simulink model "vdp_100"  (R2023b)
settings: Solver=VariableStepAuto  StartTime=0.0  StopTime=20  RelTol=1e-3  AbsTol=1e-6
libraries: simulink x100
(part 1 of 2)
Description:
  | The van der Pol Equation
  | 
  | This is a simulation of a nonlinear second order system.
settings Model: Creator=The MathWorks, Inc.  LastModifiedBy=dganesan
settings SolverCC: AutoScaleAbsTol=off  AlgebraicLoopSolver=TrustRegion
settings DataIOCC: ExternalInput=[]  InitialState=[]  SaveFormat=Array  SaveOutput=off  SaveTime=off
settings OptimizationCC: BlockReduction=off  BooleanDataType=off  ReuseModelBlockBuffer=off  InitFltsAndDblsToZero=on  LifeSpan=inf  BufferReusableBoundary=off
settings DebuggingCC: SaveWithParameterizedLinksMsg=none  SignalResolutionControl=TryResolveAllWithWarning  MultiTaskDSMMsg=warning  MultiTaskCondExecSysMsg=none  FcnCallInpInsideContextMsg=warning  UnconnectedInputMsg=warning  UnconnectedOutputMsg=warning  UnconnectedLineMsg=warning  BusObjectLabelMismatch=none  PregeneratedLibrarySubsystemCodeDiagnostic=none  SFUnexpectedBacktrackingDiag=warning  SFNoUnconditionalDefaultTransitionDiag=warning  SFExecutionAtInitializationDiag=none  ArithmeticOperatorsInVariantConditions=warning
settings HardwareCC: ProdBitPerPointer=32  ProdBitPerSizeT=32  ProdBitPerPtrDiffT=32  ProdLargestAtomicFloat=None  ProdIntDivRoundTo=Undefined  ProdEndianess=Unspecified  ProdWordSize=32  ProdHWDeviceType=32-bit Generic  TargetUnknown=on
settings ModelReferenceCC: EnableRefExpFcnMdlSchedulingChecks=on  PropagateSignalLabelsOutOfModel=off
settings SFSimCC: SimUseLocalCustomCode=off  CustomCodeUndefinedFunction=UseInterfaceOnly
settings RTWCC: RTWUseLocalCustomCode=off
settings CodeAppCC: StateflowObjectComments=on
settings GRTTargetCC: TargetFcnLib=ansi_tfl_tmw.mat  TargetLangStandard=C89/C90 (ANSI)  CombineOutputUpdateFcns=off  GRTInterface=on
settings ConfigComp: CovMetricSettings=dw  CovSaveCumulativeToWorkspaceVar=on  CovSaveSingleToWorkspaceVar=on  CovExternalEMLEnable=off

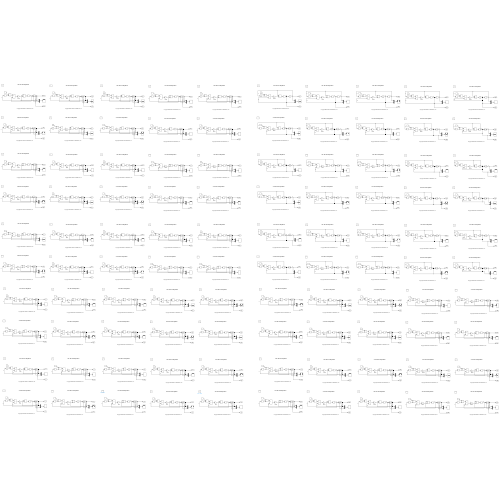
[thumbnail: Simulink's stored preview of the top-level diagram]
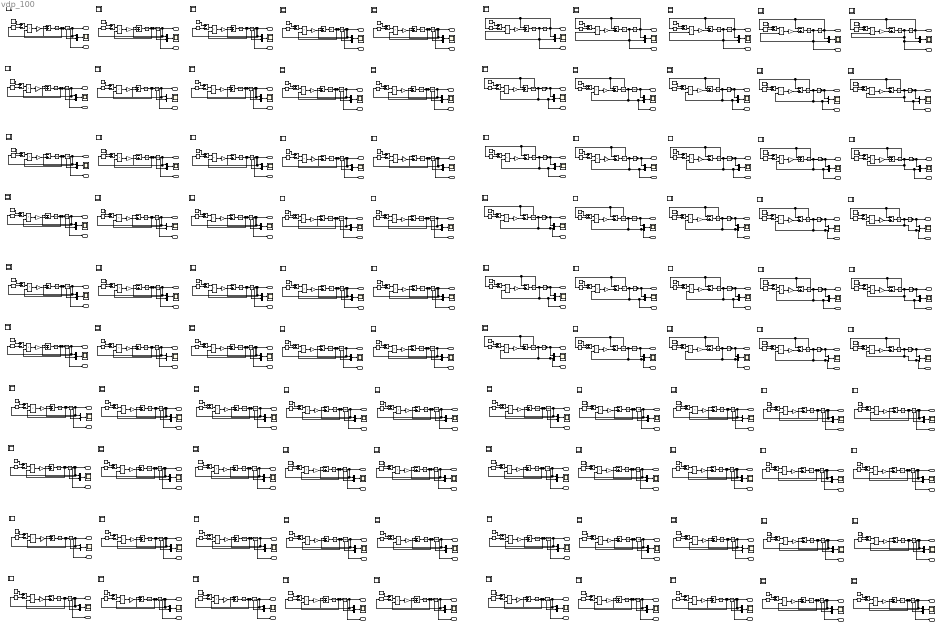
== system vdp_100 ==
  note: van der Pol Equation
  note: Copyright 2004-2020 The MathWorks, Inc.
  note: van der Pol Equation
  note: Copyright 2004-2020 The MathWorks, Inc.
  note: van der Pol Equation
  note: Copyright 2004-2020 The MathWorks, Inc.
  note: Copyright 2004-2020 The MathWorks, Inc.
  note: van der Pol Equation
  note: Copyright 2004-2020 The MathWorks, Inc.
  note: van der Pol Equation
  note: van der Pol Equation
  note: Copyright 2004-2020 The MathWorks, Inc.
  note: van der Pol Equation
  note: van der Pol Equation
  note: Copyright 2004-2020 The MathWorks, Inc.
  note: Copyright 2004-2020 The MathWorks, Inc.
  note: Copyright 2004-2020 The MathWorks, Inc.
  note: Copyright 2004-2020 The MathWorks, Inc.
  note: van der Pol Equation
  note: van der Pol Equation
  note: van der Pol Equation
  note: Copyright 2004-2020 The MathWorks, Inc.
  note: van der Pol Equation
  note: Copyright 2004-2020 The MathWorks, Inc.
  note: Copyright 2004-2020 The MathWorks, Inc.
  note: van der Pol Equation
  note: Copyright 2004-2020 The MathWorks, Inc.
  note: van der Pol Equation
  note: Copyright 2004-2020 The MathWorks, Inc.
  note: Copyright 2004-2020 The MathWorks, Inc.
  note: van der Pol Equation
  note: van der Pol Equation
  note: van der Pol Equation
  note: van der Pol Equation
  note: Copyright 2004-2020 The MathWorks, Inc.
  note: Copyright 2004-2020 The MathWorks, Inc.
  note: Copyright 2004-2020 The MathWorks, Inc.
  note: Copyright 2004-2020 The MathWorks, Inc.
  note: van der Pol Equation
  note: van der Pol Equation
  note: van der Pol Equation
  note: Copyright 2004-2020 The MathWorks, Inc.
  note: van der Pol Equation
  note: Copyright 2004-2020 The MathWorks, Inc.
  note: van der Pol Equation
  note: Copyright 2004-2020 The MathWorks, Inc.
  note: van der Pol Equation
  note: van der Pol Equation
  note: van der Pol Equation
  note: van der Pol Equation
  note: Copyright 2004-2020 The MathWorks, Inc.
  note: van der Pol Equation
  note: Copyright 2004-2020 The MathWorks, Inc.
  note: van der Pol Equation
  note: Copyright 2004-2020 The MathWorks, Inc.
  note: Copyright 2004-2020 The MathWorks, Inc.
  note: Copyright 2004-2020 The MathWorks, Inc.
  note: Copyright 2004-2020 The MathWorks, Inc.
  note: Copyright 2004-2020 The MathWorks, Inc.
  note: van der Pol Equation
  note: van der Pol Equation
  note: Copyright 2004-2020 The MathWorks, Inc.
  note: Copyright 2004-2020 The MathWorks, Inc.
  note: van der Pol Equation
  note: Copyright 2004-2020 The MathWorks, Inc.
  note: van der Pol Equation
  note: Copyright 2004-2020 The MathWorks, Inc.
  note: van der Pol Equation
  note: Copyright 2004-2020 The MathWorks, Inc.
  note: Copyright 2004-2020 The MathWorks, Inc.
  note: van der Pol Equation
  note: van der Pol Equation
  note: van der Pol Equation
  note: van der Pol Equation
  note: Copyright 2004-2020 The MathWorks, Inc.
  note: Copyright 2004-2020 The MathWorks, Inc.
  note: Copyright 2004-2020 The MathWorks, Inc.
  note: Copyright 2004-2020 The MathWorks, Inc.
  note: van der Pol Equation
  note: van der Pol Equation
  note: van der Pol Equation
  note: Copyright 2004-2020 The MathWorks, Inc.
  note: Copyright 2004-2020 The MathWorks, Inc.
  note: Copyright 2004-2020 The MathWorks, Inc.
  note: van der Pol Equation
  note: Copyright 2004-2020 The MathWorks, Inc.
  note: van der Pol Equation
  note: Copyright 2004-2020 The MathWorks, Inc.
  note: van der Pol Equation
  note: Copyright 2004-2020 The MathWorks, Inc.
  note: Copyright 2004-2020 The MathWorks, Inc.
  note: van der Pol Equation
  note: van der Pol Equation
  note: Copyright 2004-2020 The MathWorks, Inc.
  note: Copyright 2004-2020 The MathWorks, Inc.
  note: Copyright 2004-2020 The MathWorks, Inc.
  note: van der Pol Equation
  note: van der Pol Equation
  note: van der Pol Equation
  note: van der Pol Equation
  note: Copyright 2004-2020 The MathWorks, Inc.
  note: van der Pol Equation
  note: van der Pol Equation
  note: Copyright 2004-2020 The MathWorks, Inc.
  note: van der Pol Equation
  note: Copyright 2004-2020 The MathWorks, Inc.
  note: Copyright 2004-2020 The MathWorks, Inc.
  note: Copyright 2004-2020 The MathWorks, Inc.
  note: Copyright 2004-2020 The MathWorks, Inc.
  note: van der Pol Equation
  note: van der Pol Equation
  note: Copyright 2004-2020 The MathWorks, Inc.
  note: van der Pol Equation
  note: van der Pol Equation
  note: Copyright 2004-2020 The MathWorks, Inc.
  note: van der Pol Equation
  note: Copyright 2004-2020 The MathWorks, Inc.
  note: van der Pol Equation
  note: Copyright 2004-2020 The MathWorks, Inc.
  note: van der Pol Equation
  note: van der Pol Equation
  note: van der Pol Equation
  note: Copyright 2004-2020 The MathWorks, Inc.
  note: van der Pol Equation
  note: van der Pol Equation
  note: Copyright 2004-2020 The MathWorks, Inc.
  note: Copyright 2004-2020 The MathWorks, Inc.
  note: Copyright 2004-2020 The MathWorks, Inc.
  note: van der Pol Equation
  note: van der Pol Equation
  note: van der Pol Equation
  note: Copyright 2004-2020 The MathWorks, Inc.
  note: Copyright 2004-2020 The MathWorks, Inc.
  note: Copyright 2004-2020 The MathWorks, Inc.
  note: Copyright 2004-2020 The MathWorks, Inc.
  note: van der Pol Equation
  note: Copyright 2004-2020 The MathWorks, Inc.
  note: Copyright 2004-2020 The MathWorks, Inc.
  note: Copyright 2004-2020 The MathWorks, Inc.
  note: van der Pol Equation
  note: van der Pol Equation
  note: van der Pol Equation
  note: Copyright 2004-2020 The MathWorks, Inc.
  note: van der Pol Equation
  note: van der Pol Equation
  note: van der Pol Equation
  note: van der Pol Equation
  note: Copyright 2004-2020 The MathWorks, Inc.
  note: Copyright 2004-2020 The MathWorks, Inc.
  note: van der Pol Equation
  note: van der Pol Equation
  note: Copyright 2004-2020 The MathWorks, Inc.
  note: van der Pol Equation
  note: Copyright 2004-2020 The MathWorks, Inc.
  note: van der Pol Equation
  note: van der Pol Equation
  note: van der Pol Equation
  note: van der Pol Equation
  note: van der Pol Equation
  note: Copyright 2004-2020 The MathWorks, Inc.
  note: Copyright 2004-2020 The MathWorks, Inc.
  note: van der Pol Equation
  note: Copyright 2004-2020 The MathWorks, Inc.
  note: van der Pol Equation
  note: Copyright 2004-2020 The MathWorks, Inc.
  note: Copyright 2004-2020 The MathWorks, Inc.
  note: Copyright 2004-2020 The MathWorks, Inc.
  note: Copyright 2004-2020 The MathWorks, Inc.
  note: Copyright 2004-2020 The MathWorks, Inc.
  note: van der Pol Equation
  note: Copyright 2004-2020 The MathWorks, Inc.
  note: Copyright 2004-2020 The MathWorks, Inc.
  note: van der Pol Equation
  note: Copyright 2004-2020 The MathWorks, Inc.
  note: van der Pol Equation
  note: Copyright 2004-2020 The MathWorks, Inc.
  note: van der Pol Equation
  note: van der Pol Equation
  note: van der Pol Equation
  note: Copyright 2004-2020 The MathWorks, Inc.
  note: van der Pol Equation
  note: Copyright 2004-2020 The MathWorks, Inc.
  note: Copyright 2004-2020 The MathWorks, Inc.
  note: van der Pol Equation
  note: Copyright 2004-2020 The MathWorks, Inc.
  note: Copyright 2004-2020 The MathWorks, Inc.
  note: van der Pol Equation
  note: Copyright 2004-2020 The MathWorks, Inc.
  note: van der Pol Equation
  note: van der Pol Equation
  note: van der Pol Equation
  note: Copyright 2004-2020 The MathWorks, Inc.
  note: Copyright 2004-2020 The MathWorks, Inc.
  note: Copyright 2004-2020 The MathWorks, Inc.
  note: van der Pol Equation
  note: Copyright 2004-2020 The MathWorks, Inc.
  note: Copyright 2004-2020 The MathWorks, Inc.
  note: Copyright 2004-2020 The MathWorks, Inc.
  note: van der Pol Equation
  note: van der Pol Equation
  Constant{,1..99} (100 alike) : Constant
  More Info : Subsystem
      mask Display: disp('?')
  More Info1 : Subsystem
      mask Display: disp('?')
  More Info10 : Subsystem
      mask Display: disp('?')
  More Info11 : Subsystem
      mask Display: disp('?')
  More Info12 : Subsystem
      mask Display: disp('?')
  More Info13 : Subsystem
      mask Display: disp('?')
  More Info14 : Subsystem
      mask Display: disp('?')
  More Info15 : Subsystem
      mask Display: disp('?')
  More Info16 : Subsystem
      mask Display: disp('?')
  More Info17 : Subsystem
      mask Display: disp('?')
  More Info18 : Subsystem
      mask Display: disp('?')
  More Info19 : Subsystem
      mask Display: disp('?')
  More Info2 : Subsystem
      mask Display: disp('?')
  More Info20 : Subsystem
      mask Display: disp('?')
  More Info21 : Subsystem
      mask Display: disp('?')
  More Info22 : Subsystem
      mask Display: disp('?')
  More Info23 : Subsystem
      mask Display: disp('?')
  More Info24 : Subsystem
      mask Display: disp('?')
  More Info25 : Subsystem
      mask Display: disp('?')
  More Info26 : Subsystem
      mask Display: disp('?')
  More Info27 : Subsystem
      mask Display: disp('?')
  More Info28 : Subsystem
      mask Display: disp('?')
  More Info29 : Subsystem
      mask Display: disp('?')
  More Info3 : Subsystem
      mask Display: disp('?')
  More Info30 : Subsystem
      mask Display: disp('?')
  More Info31 : Subsystem
      mask Display: disp('?')
  More Info32 : Subsystem
      mask Display: disp('?')
  More Info33 : Subsystem
      mask Display: disp('?')
  More Info34 : Subsystem
      mask Display: disp('?')
  More Info35 : Subsystem
      mask Display: disp('?')
  More Info36 : Subsystem
      mask Display: disp('?')
  More Info37 : Subsystem
      mask Display: disp('?')
  More Info38 : Subsystem
      mask Display: disp('?')
  More Info39 : Subsystem
      mask Display: disp('?')
  More Info4 : Subsystem
      mask Display: disp('?')
  More Info40 : Subsystem
      mask Display: disp('?')
  More Info41 : Subsystem
      mask Display: disp('?')
  More Info42 : Subsystem
      mask Display: disp('?')
  More Info43 : Subsystem
      mask Display: disp('?')
  More Info44 : Subsystem
      mask Display: disp('?')
  More Info45 : Subsystem
      mask Display: disp('?')
  More Info46 : Subsystem
      mask Display: disp('?')
  More Info47 : Subsystem
      mask Display: disp('?')
  More Info48 : Subsystem
      mask Display: disp('?')
  More Info49 : Subsystem
      mask Display: disp('?')
  More Info5 : Subsystem
      mask Display: disp('?')
  More Info50 : Subsystem
      mask Display: disp('?')
  More Info51 : Subsystem
      mask Display: disp('?')
  More Info52 : Subsystem
      mask Display: disp('?')
  More Info53 : Subsystem
      mask Display: disp('?')
  More Info54 : Subsystem
      mask Display: disp('?')
  More Info55 : Subsystem
      mask Display: disp('?')
  More Info56 : Subsystem
      mask Display: disp('?')
  More Info57 : Subsystem
      mask Display: disp('?')
  More Info58 : Subsystem
      mask Display: disp('?')
  More Info59 : Subsystem
      mask Display: disp('?')
  More Info6 : Subsystem
      mask Display: disp('?')
  More Info60 : Subsystem
      mask Display: disp('?')
  More Info61 : Subsystem
      mask Display: disp('?')
  More Info62 : Subsystem
      mask Display: disp('?')
  More Info63 : Subsystem
      mask Display: disp('?')
  More Info64 : Subsystem
      mask Display: disp('?')
  More Info65 : Subsystem
      mask Display: disp('?')
  More Info66 : Subsystem
      mask Display: disp('?')
  More Info67 : Subsystem
      mask Display: disp('?')
  More Info68 : Subsystem
      mask Display: disp('?')
  More Info69 : Subsystem
      mask Display: disp('?')
  More Info7 : Subsystem
      mask Display: disp('?')
  More Info70 : Subsystem
      mask Display: disp('?')
  More Info71 : Subsystem
      mask Display: disp('?')
  More Info72 : Subsystem
      mask Display: disp('?')
  More Info73 : Subsystem
      mask Display: disp('?')
  More Info74 : Subsystem
      mask Display: disp('?')
  More Info75 : Subsystem
      mask Display: disp('?')
  More Info76 : Subsystem
      mask Display: disp('?')
  More Info77 : Subsystem
      mask Display: disp('?')
  More Info78 : Subsystem
      mask Display: disp('?')
  More Info79 : Subsystem
      mask Display: disp('?')
  More Info8 : Subsystem
      mask Display: disp('?')
  More Info80 : Subsystem
      mask Display: disp('?')
  More Info81 : Subsystem
      mask Display: disp('?')
  More Info82 : Subsystem
      mask Display: disp('?')
  More Info83 : Subsystem
      mask Display: disp('?')
  More Info84 : Subsystem
      mask Display: disp('?')
  More Info85 : Subsystem
      mask Display: disp('?')
  More Info86 : Subsystem
      mask Display: disp('?')
  More Info87 : Subsystem
      mask Display: disp('?')
  More Info88 : Subsystem
      mask Display: disp('?')
  More Info89 : Subsystem
      mask Display: disp('?')
  More Info9 : Subsystem
      mask Display: disp('?')
  More Info90 : Subsystem
      mask Display: disp('?')
  More Info91 : Subsystem
      mask Display: disp('?')
  More Info92 : Subsystem
      mask Display: disp('?')
  More Info93 : Subsystem
      mask Display: disp('?')
  More Info94 : Subsystem
      mask Display: disp('?')
  More Info95 : Subsystem
      mask Display: disp('?')
  More Info96 : Subsystem
      mask Display: disp('?')
  More Info97 : Subsystem
      mask Display: disp('?')
  More Info98 : Subsystem
      mask Display: disp('?')
  More Info99 : Subsystem
      mask Display: disp('?')
  Mu{,1..99} (100 alike) : Gain  SaturateOnIntegerOverflow=on  OutDataTypeStr=Inherit: Same as input  ParamDataTypeStr=Inherit: Same as input
  Mux{,1..99} (100 alike) : Mux  Inputs=2
  Product{,1..99} (100 alike) : Product  InputSameDT=on  RndMeth=Zero  SaturateOnIntegerOverflow=on  OutDataTypeStr=Inherit: Same as first input
  Scope{,1..99} (100 alike) : Scope
  Square{,1..99} (100 alike) : Math  Operator=square
  Sum{,2,4,6,8,10,12,14,16,18,20,22,24,26,28,30,32,34,36,38,40,42,44,46,48,50,52..53,55,57,59,61,64,66,68,70,72,74,76,78,80,82,84,86,88,90,92,94,96,98,100,102,104,106,108,110,112..113,115,117,119,121,124,126,128,130,132,134..135,137,139,141,143,146,148..149,151,153,155..156,158,161,163,165,168,170,172,174,176,178..179,181,183,185,187,190,192,194,196,198} (100 alike) : Sum  Inputs=-+  InputSameDT=on  SaturateOnIntegerOverflow=on  OutDataTypeStr=Inherit: Same as first input
  Sum{1,3,5,7,9,11,13,15,17,19,21,23,25,27,29,31,33,35,37,39,41,43,45,47,49,51,54,56,58,60,62..63,65,67,69,71,73,75,77,79,81,83,85,87,89,91,93,95,97,99,101,103,105,107,109,111,114,116,118,120,122..123,125,127,129,131,133,136,138,140,142,144..145,147,150,152,154,157,159..160,162,164,166..167,169,171,173,175,177,180,182,184,186,188..189,191,193,195,197,199} (100 alike) : Sum  Inputs=+-  InputSameDT=on  SaturateOnIntegerOverflow=on  OutDataTypeStr=Inherit: Same as first input
  x{1,3,5,7,9,11,14,16,18,20..21,23,26,28,30,33..34,36,38,40..41,43,46,48,50,53..54,56,59,61,63..64,67..68,70,72,75..76,78,80..81,83,86,88,90,93..94,96,98,100..101,103..104,107,109,111,114..115,117,120,122,124..125,128..129,131,133,136..137,139,142,144,146..147,150..151,153,156,159,161..162,165..166,168..169,171,174..175,177,180..181,183,186,188,190..191,194..195,197,199} (100 alike) : Integrator  InitialCondition=2
  x{2,4,6,8,10,12..13,15,17,19,22,24..25,27,29,31..32,35,37,39,42,44..45,47,49,51..52,55,57..58,60,62,65..66,69,71,73..74,77,79,82,84..85,87,89,91..92,95,97,99,102,105..106,108,110,112..113,116,118..119,121,123,126..127,130,132,134..135,138,140..141,143,145,148..149,152,154..155,157..158,160,163..164,167,170,172..173,176,178..179,182,184..185,187,189,192..193,196,198,200} (100 alike) : Integrator
  Out1 : Outport  InitialOutput=0  VectorParamsAs1DForOutWhenUnconnected=off
  Out2 : Outport  Port=2  InitialOutput=0  VectorParamsAs1DForOutWhenUnconnected=off
  Out3 : Outport  Port=3  InitialOutput=0  VectorParamsAs1DForOutWhenUnconnected=off
  Out4 : Outport  Port=4  InitialOutput=0  VectorParamsAs1DForOutWhenUnconnected=off
  Out5 : Outport  Port=5  InitialOutput=0  VectorParamsAs1DForOutWhenUnconnected=off
  Out6 : Outport  Port=6  InitialOutput=0  VectorParamsAs1DForOutWhenUnconnected=off
  Out7 : Outport  Port=7  InitialOutput=0  VectorParamsAs1DForOutWhenUnconnected=off
  Out8 : Outport  Port=8  InitialOutput=0  VectorParamsAs1DForOutWhenUnconnected=off
  Out9 : Outport  Port=9  InitialOutput=0  VectorParamsAs1DForOutWhenUnconnected=off
  Out10 : Outport  Port=10  InitialOutput=0  VectorParamsAs1DForOutWhenUnconnected=off
  Out11 : Outport  Port=11  InitialOutput=0  VectorParamsAs1DForOutWhenUnconnected=off
  Out12 : Outport  Port=12  InitialOutput=0  VectorParamsAs1DForOutWhenUnconnected=off
  Out13 : Outport  Port=13  InitialOutput=0  VectorParamsAs1DForOutWhenUnconnected=off
  Out14 : Outport  Port=14  InitialOutput=0  VectorParamsAs1DForOutWhenUnconnected=off
  Out15 : Outport  Port=15  InitialOutput=0  VectorParamsAs1DForOutWhenUnconnected=off
  Out16 : Outport  Port=16  InitialOutput=0  VectorParamsAs1DForOutWhenUnconnected=off
  Out17 : Outport  Port=17  InitialOutput=0  VectorParamsAs1DForOutWhenUnconnected=off
  Out18 : Outport  Port=18  InitialOutput=0  VectorParamsAs1DForOutWhenUnconnected=off
  Out19 : Outport  Port=19  InitialOutput=0  VectorParamsAs1DForOutWhenUnconnected=off
  Out20 : Outport  Port=20  InitialOutput=0  VectorParamsAs1DForOutWhenUnconnected=off
  Out21 : Outport  Port=21  InitialOutput=0  VectorParamsAs1DForOutWhenUnconnected=off
  Out22 : Outport  Port=22  InitialOutput=0  VectorParamsAs1DForOutWhenUnconnected=off
  Out23 : Outport  Port=23  InitialOutput=0  VectorParamsAs1DForOutWhenUnconnected=off
  Out24 : Outport  Port=24  InitialOutput=0  VectorParamsAs1DForOutWhenUnconnected=off
  Out25 : Outport  Port=25  InitialOutput=0  VectorParamsAs1DForOutWhenUnconnected=off
  Out26 : Outport  Port=26  InitialOutput=0  VectorParamsAs1DForOutWhenUnconnected=off
  Out27 : Outport  Port=27  InitialOutput=0  VectorParamsAs1DForOutWhenUnconnected=off
  Out28 : Outport  Port=28  InitialOutput=0  VectorParamsAs1DForOutWhenUnconnected=off
  Out29 : Outport  Port=29  InitialOutput=0  VectorParamsAs1DForOutWhenUnconnected=off
  Out30 : Outport  Port=30  InitialOutput=0  VectorParamsAs1DForOutWhenUnconnected=off
  Out31 : Outport  Port=31  InitialOutput=0  VectorParamsAs1DForOutWhenUnconnected=off
  Out32 : Outport  Port=32  InitialOutput=0  VectorParamsAs1DForOutWhenUnconnected=off
  Out33 : Outport  Port=33  InitialOutput=0  VectorParamsAs1DForOutWhenUnconnected=off
  Out34 : Outport  Port=34  InitialOutput=0  VectorParamsAs1DForOutWhenUnconnected=off
  Out35 : Outport  Port=35  InitialOutput=0  VectorParamsAs1DForOutWhenUnconnected=off
  Out36 : Outport  Port=36  InitialOutput=0  VectorParamsAs1DForOutWhenUnconnected=off
  Out37 : Outport  Port=37  InitialOutput=0  VectorParamsAs1DForOutWhenUnconnected=off
  Out38 : Outport  Port=38  InitialOutput=0  VectorParamsAs1DForOutWhenUnconnected=off
  Out39 : Outport  Port=39  InitialOutput=0  VectorParamsAs1DForOutWhenUnconnected=off
  Out40 : Outport  Port=40  InitialOutput=0  VectorParamsAs1DForOutWhenUnconnected=off
  Out41 : Outport  Port=41  InitialOutput=0  VectorParamsAs1DForOutWhenUnconnected=off
  Out42 : Outport  Port=42  InitialOutput=0  VectorParamsAs1DForOutWhenUnconnected=off
  Out43 : Outport  Port=43  InitialOutput=0  VectorParamsAs1DForOutWhenUnconnected=off
  Out44 : Outport  Port=44  InitialOutput=0  VectorParamsAs1DForOutWhenUnconnected=off
  Out45 : Outport  Port=45  InitialOutput=0  VectorParamsAs1DForOutWhenUnconnected=off
  Out46 : Outport  Port=46  InitialOutput=0  VectorParamsAs1DForOutWhenUnconnected=off
  Out47 : Outport  Port=47  InitialOutput=0  VectorParamsAs1DForOutWhenUnconnected=off
  Out48 : Outport  Port=48  InitialOutput=0  VectorParamsAs1DForOutWhenUnconnected=off
  Out49 : Outport  Port=49  InitialOutput=0  VectorParamsAs1DForOutWhenUnconnected=off
  Out50 : Outport  Port=50  InitialOutput=0  VectorParamsAs1DForOutWhenUnconnected=off
  Out51 : Outport  Port=51  InitialOutput=0  VectorParamsAs1DForOutWhenUnconnected=off
  Out52 : Outport  Port=52  InitialOutput=0  VectorParamsAs1DForOutWhenUnconnected=off
  Out53 : Outport  Port=53  InitialOutput=0  VectorParamsAs1DForOutWhenUnconnected=off
  Out54 : Outport  Port=54  InitialOutput=0  VectorParamsAs1DForOutWhenUnconnected=off
  Out55 : Outport  Port=55  InitialOutput=0  VectorParamsAs1DForOutWhenUnconnected=off
  Out56 : Outport  Port=56  InitialOutput=0  VectorParamsAs1DForOutWhenUnconnected=off
  Out57 : Outport  Port=57  InitialOutput=0  VectorParamsAs1DForOutWhenUnconnected=off
  Out58 : Outport  Port=58  InitialOutput=0  VectorParamsAs1DForOutWhenUnconnected=off
  Out59 : Outport  Port=59  InitialOutput=0  VectorParamsAs1DForOutWhenUnconnected=off
  Out60 : Outport  Port=60  InitialOutput=0  VectorParamsAs1DForOutWhenUnconnected=off
  Out61 : Outport  Port=61  InitialOutput=0  VectorParamsAs1DForOutWhenUnconnected=off
  Out62 : Outport  Port=62  InitialOutput=0  VectorParamsAs1DForOutWhenUnconnected=off
  Out63 : Outport  Port=63  InitialOutput=0  VectorParamsAs1DForOutWhenUnconnected=off
  Out64 : Outport  Port=64  InitialOutput=0  VectorParamsAs1DForOutWhenUnconnected=off
  Out65 : Outport  Port=65  InitialOutput=0  VectorParamsAs1DForOutWhenUnconnected=off
  Out66 : Outport  Port=66  InitialOutput=0  VectorParamsAs1DForOutWhenUnconnected=off
  Out67 : Outport  Port=67  InitialOutput=0  VectorParamsAs1DForOutWhenUnconnected=off
  Out68 : Outport  Port=68  InitialOutput=0  VectorParamsAs1DForOutWhenUnconnected=off
  Out69 : Outport  Port=69  InitialOutput=0  VectorParamsAs1DForOutWhenUnconnected=off
  Out70 : Outport  Port=70  InitialOutput=0  VectorParamsAs1DForOutWhenUnconnected=off
  Out71 : Outport  Port=71  InitialOutput=0  VectorParamsAs1DForOutWhenUnconnected=off
  Out72 : Outport  Port=72  InitialOutput=0  VectorParamsAs1DForOutWhenUnconnected=off
  Out73 : Outport  Port=73  InitialOutput=0  VectorParamsAs1DForOutWhenUnconnected=off
  Out74 : Outport  Port=74  InitialOutput=0  VectorParamsAs1DForOutWhenUnconnected=off
  Out75 : Outport  Port=75  InitialOutput=0  VectorParamsAs1DForOutWhenUnconnected=off
  Out76 : Outport  Port=76  InitialOutput=0  VectorParamsAs1DForOutWhenUnconnected=off
  Out77 : Outport  Port=77  InitialOutput=0  VectorParamsAs1DForOutWhenUnconnected=off
  Out78 : Outport  Port=78  InitialOutput=0  VectorParamsAs1DForOutWhenUnconnected=off
  Out79 : Outport  Port=79  InitialOutput=0  VectorParamsAs1DForOutWhenUnconnected=off
  Out80 : Outport  Port=80  InitialOutput=0  VectorParamsAs1DForOutWhenUnconnected=off
  Out81 : Outport  Port=81  InitialOutput=0  VectorParamsAs1DForOutWhenUnconnected=off
  Out82 : Outport  Port=82  InitialOutput=0  VectorParamsAs1DForOutWhenUnconnected=off
  Out83 : Outport  Port=83  InitialOutput=0  VectorParamsAs1DForOutWhenUnconnected=off
  Out84 : Outport  Port=84  InitialOutput=0  VectorParamsAs1DForOutWhenUnconnected=off
  Out85 : Outport  Port=85  InitialOutput=0  VectorParamsAs1DForOutWhenUnconnected=off
  Out86 : Outport  Port=86  InitialOutput=0  VectorParamsAs1DForOutWhenUnconnected=off
  Out87 : Outport  Port=87  InitialOutput=0  VectorParamsAs1DForOutWhenUnconnected=off
  Out88 : Outport  Port=88  InitialOutput=0  VectorParamsAs1DForOutWhenUnconnected=off
  Out89 : Outport  Port=89  InitialOutput=0  VectorParamsAs1DForOutWhenUnconnected=off
  Out90 : Outport  Port=90  InitialOutput=0  VectorParamsAs1DForOutWhenUnconnected=off
  Out91 : Outport  Port=91  InitialOutput=0  VectorParamsAs1DForOutWhenUnconnected=off
  Out92 : Outport  Port=92  InitialOutput=0  VectorParamsAs1DForOutWhenUnconnected=off
  Out93 : Outport  Port=93  InitialOutput=0  VectorParamsAs1DForOutWhenUnconnected=off
  Out94 : Outport  Port=94  InitialOutput=0  VectorParamsAs1DForOutWhenUnconnected=off
  Out95 : Outport  Port=95  InitialOutput=0  VectorParamsAs1DForOutWhenUnconnected=off
  Out96 : Outport  Port=96  InitialOutput=0  VectorParamsAs1DForOutWhenUnconnected=off
  Out97 : Outport  Port=97  InitialOutput=0  VectorParamsAs1DForOutWhenUnconnected=off
  Out98 : Outport  Port=98  InitialOutput=0  VectorParamsAs1DForOutWhenUnconnected=off
  Out99 : Outport  Port=99  InitialOutput=0  VectorParamsAs1DForOutWhenUnconnected=off
  Out100 : Outport  Port=100  InitialOutput=0  VectorParamsAs1DForOutWhenUnconnected=off
  Out101 : Outport  Port=101  InitialOutput=0  VectorParamsAs1DForOutWhenUnconnected=off
  Out102 : Outport  Port=102  InitialOutput=0  VectorParamsAs1DForOutWhenUnconnected=off
  Out103 : Outport  Port=103  InitialOutput=0  VectorParamsAs1DForOutWhenUnconnected=off
  Out104 : Outport  Port=104  InitialOutput=0  VectorParamsAs1DForOutWhenUnconnected=off
  Out105 : Outport  Port=105  InitialOutput=0  VectorParamsAs1DForOutWhenUnconnected=off
  Out106 : Outport  Port=106  InitialOutput=0  VectorParamsAs1DForOutWhenUnconnected=off
  Out107 : Outport  Port=107  InitialOutput=0  VectorParamsAs1DForOutWhenUnconnected=off
  Out108 : Outport  Port=108  InitialOutput=0  VectorParamsAs1DForOutWhenUnconnected=off
  Out109 : Outport  Port=109  InitialOutput=0  VectorParamsAs1DForOutWhenUnconnected=off
  Out110 : Outport  Port=110  InitialOutput=0  VectorParamsAs1DForOutWhenUnconnected=off
  Out111 : Outport  Port=111  InitialOutput=0  VectorParamsAs1DForOutWhenUnconnected=off
  Out112 : Outport  Port=112  InitialOutput=0  VectorParamsAs1DForOutWhenUnconnected=off
  Out113 : Outport  Port=113  InitialOutput=0  VectorParamsAs1DForOutWhenUnconnected=off
  Out114 : Outport  Port=114  InitialOutput=0  VectorParamsAs1DForOutWhenUnconnected=off
  Out115 : Outport  Port=115  InitialOutput=0  VectorParamsAs1DForOutWhenUnconnected=off
  Out116 : Outport  Port=116  InitialOutput=0  VectorParamsAs1DForOutWhenUnconnected=off
  Out117 : Outport  Port=117  InitialOutput=0  VectorParamsAs1DForOutWhenUnconnected=off
  Out118 : Outport  Port=118  InitialOutput=0  VectorParamsAs1DForOutWhenUnconnected=off
  Out119 : Outport  Port=119  InitialOutput=0  VectorParamsAs1DForOutWhenUnconnected=off
  Out120 : Outport  Port=120  InitialOutput=0  VectorParamsAs1DForOutWhenUnconnected=off
  Out121 : Outport  Port=121  InitialOutput=0  VectorParamsAs1DForOutWhenUnconnected=off
  Out122 : Outport  Port=122  InitialOutput=0  VectorParamsAs1DForOutWhenUnconnected=off
  Out123 : Outport  Port=123  InitialOutput=0  VectorParamsAs1DForOutWhenUnconnected=off
  Out124 : Outport  Port=124  InitialOutput=0  VectorParamsAs1DForOutWhenUnconnected=off
  Out125 : Outport  Port=125  InitialOutput=0  VectorParamsAs1DForOutWhenUnconnected=off
  Out126 : Outport  Port=126  InitialOutput=0  VectorParamsAs1DForOutWhenUnconnected=off
  Out127 : Outport  Port=127  InitialOutput=0  VectorParamsAs1DForOutWhenUnconnected=off
  Out128 : Outport  Port=128  InitialOutput=0  VectorParamsAs1DForOutWhenUnconnected=off
  Out129 : Outport  Port=129  InitialOutput=0  VectorParamsAs1DForOutWhenUnconnected=off
  Out130 : Outport  Port=130  InitialOutput=0  VectorParamsAs1DForOutWhenUnconnected=off
  Out131 : Outport  Port=131  InitialOutput=0  VectorParamsAs1DForOutWhenUnconnected=off
  Out132 : Outport  Port=132  InitialOutput=0  VectorParamsAs1DForOutWhenUnconnected=off
  Out133 : Outport  Port=133  InitialOutput=0  VectorParamsAs1DForOutWhenUnconnected=off
  Out134 : Outport  Port=134  InitialOutput=0  VectorParamsAs1DForOutWhenUnconnected=off
  Out135 : Outport  Port=135  InitialOutput=0  VectorParamsAs1DForOutWhenUnconnected=off
  Out136 : Outport  Port=136  InitialOutput=0  VectorParamsAs1DForOutWhenUnconnected=off
  Out137 : Outport  Port=137  InitialOutput=0  VectorParamsAs1DForOutWhenUnconnected=off
  Out138 : Outport  Port=138  InitialOutput=0  VectorParamsAs1DForOutWhenUnconnected=off
  Out139 : Outport  Port=139  InitialOutput=0  VectorParamsAs1DForOutWhenUnconnected=off
  Out140 : Outport  Port=140  InitialOutput=0  VectorParamsAs1DForOutWhenUnconnected=off
  Out141 : Outport  Port=141  InitialOutput=0  VectorParamsAs1DForOutWhenUnconnected=off
  Out142 : Outport  Port=142  InitialOutput=0  VectorParamsAs1DForOutWhenUnconnected=off
  Out143 : Outport  Port=143  InitialOutput=0  VectorParamsAs1DForOutWhenUnconnected=off
  Out144 : Outport  Port=144  InitialOutput=0  VectorParamsAs1DForOutWhenUnconnected=off
  Out145 : Outport  Port=145  InitialOutput=0  VectorParamsAs1DForOutWhenUnconnected=off
  Out146 : Outport  Port=146  InitialOutput=0  VectorParamsAs1DForOutWhenUnconnected=off
  Out147 : Outport  Port=147  InitialOutput=0  VectorParamsAs1DForOutWhenUnconnected=off
  Out148 : Outport  Port=148  InitialOutput=0  VectorParamsAs1DForOutWhenUnconnected=off
  Out149 : Outport  Port=149  InitialOutput=0  VectorParamsAs1DForOutWhenUnconnected=off
  Out150 : Outport  Port=150  InitialOutput=0  VectorParamsAs1DForOutWhenUnconnected=off
  Out151 : Outport  Port=151  InitialOutput=0  VectorParamsAs1DForOutWhenUnconnected=off
  Out152 : Outport  Port=152  InitialOutput=0  VectorParamsAs1DForOutWhenUnconnected=off
  Out153 : Outport  Port=153  InitialOutput=0  VectorParamsAs1DForOutWhenUnconnected=off
  Out154 : Outport  Port=154  InitialOutput=0  VectorParamsAs1DForOutWhenUnconnected=off
  Out155 : Outport  Port=155  InitialOutput=0  VectorParamsAs1DForOutWhenUnconnected=off
  Out156 : Outport  Port=156  InitialOutput=0  VectorParamsAs1DForOutWhenUnconnected=off
  Out157 : Outport  Port=157  InitialOutput=0  VectorParamsAs1DForOutWhenUnconnected=off
  Out158 : Outport  Port=158  InitialOutput=0  VectorParamsAs1DForOutWhenUnconnected=off
  Out159 : Outport  Port=159  InitialOutput=0  VectorParamsAs1DForOutWhenUnconnected=off
  Out160 : Outport  Port=160  InitialOutput=0  VectorParamsAs1DForOutWhenUnconnected=off
  Out161 : Outport  Port=161  InitialOutput=0  VectorParamsAs1DForOutWhenUnconnected=off
  Out162 : Outport  Port=162  InitialOutput=0  VectorParamsAs1DForOutWhenUnconnected=off
  Out163 : Outport  Port=163  InitialOutput=0  VectorParamsAs1DForOutWhenUnconnected=off
  Out164 : Outport  Port=164  InitialOutput=0  VectorParamsAs1DForOutWhenUnconnected=off
  Out165 : Outport  Port=165  InitialOutput=0  VectorParamsAs1DForOutWhenUnconnected=off
  Out166 : Outport  Port=166  InitialOutput=0  VectorParamsAs1DForOutWhenUnconnected=off
  Out167 : Outport  Port=167  InitialOutput=0  VectorParamsAs1DForOutWhenUnconnected=off
  Out168 : Outport  Port=168  InitialOutput=0  VectorParamsAs1DForOutWhenUnconnected=off
  Out169 : Outport  Port=169  InitialOutput=0  VectorParamsAs1DForOutWhenUnconnected=off
  Out170 : Outport  Port=170  InitialOutput=0  VectorParamsAs1DForOutWhenUnconnected=off
  Out171 : Outport  Port=171  InitialOutput=0  VectorParamsAs1DForOutWhenUnconnected=off
  Out172 : Outport  Port=172  InitialOutput=0  VectorParamsAs1DForOutWhenUnconnected=off
  Out173 : Outport  Port=173  InitialOutput=0  VectorParamsAs1DForOutWhenUnconnected=off
  Out174 : Outport  Port=174  InitialOutput=0  VectorParamsAs1DForOutWhenUnconnected=off
  Out175 : Outport  Port=175  InitialOutput=0  VectorParamsAs1DForOutWhenUnconnected=off
  Out176 : Outport  Port=176  InitialOutput=0  VectorParamsAs1DForOutWhenUnconnected=off
  Out177 : Outport  Port=177  InitialOutput=0  VectorParamsAs1DForOutWhenUnconnected=off
  Out178 : Outport  Port=178  InitialOutput=0  VectorParamsAs1DForOutWhenUnconnected=off
  Out179 : Outport  Port=179  InitialOutput=0  VectorParamsAs1DForOutWhenUnconnected=off
  Out180 : Outport  Port=180  InitialOutput=0  VectorParamsAs1DForOutWhenUnconnected=off
  Out181 : Outport  Port=181  InitialOutput=0  VectorParamsAs1DForOutWhenUnconnected=off
  Out182 : Outport  Port=182  InitialOutput=0  VectorParamsAs1DForOutWhenUnconnected=off
  Out183 : Outport  Port=183  InitialOutput=0  VectorParamsAs1DForOutWhenUnconnected=off
  Out184 : Outport  Port=184  InitialOutput=0  VectorParamsAs1DForOutWhenUnconnected=off
  Out185 : Outport  Port=185  InitialOutput=0  VectorParamsAs1DForOutWhenUnconnected=off
  Out186 : Outport  Port=186  InitialOutput=0  VectorParamsAs1DForOutWhenUnconnected=off
  Out187 : Outport  Port=187  InitialOutput=0  VectorParamsAs1DForOutWhenUnconnected=off
  Out188 : Outport  Port=188  InitialOutput=0  VectorParamsAs1DForOutWhenUnconnected=off
  Out189 : Outport  Port=189  InitialOutput=0  VectorParamsAs1DForOutWhenUnconnected=off
  Out190 : Outport  Port=190  InitialOutput=0  VectorParamsAs1DForOutWhenUnconnected=off
  Out191 : Outport  Port=191  InitialOutput=0  VectorParamsAs1DForOutWhenUnconnected=off
  Out192 : Outport  Port=192  InitialOutput=0  VectorParamsAs1DForOutWhenUnconnected=off
  Out193 : Outport  Port=193  InitialOutput=0  VectorParamsAs1DForOutWhenUnconnected=off
  Out194 : Outport  Port=194  InitialOutput=0  VectorParamsAs1DForOutWhenUnconnected=off
  Out195 : Outport  Port=195  InitialOutput=0  VectorParamsAs1DForOutWhenUnconnected=off
  Out196 : Outport  Port=196  InitialOutput=0  VectorParamsAs1DForOutWhenUnconnected=off
  Out197 : Outport  Port=197  InitialOutput=0  VectorParamsAs1DForOutWhenUnconnected=off
  Out198 : Outport  Port=198  InitialOutput=0  VectorParamsAs1DForOutWhenUnconnected=off
  Out199 : Outport  Port=199  InitialOutput=0  VectorParamsAs1DForOutWhenUnconnected=off
  Out200 : Outport  Port=200  InitialOutput=0  VectorParamsAs1DForOutWhenUnconnected=off
  wires:
  Sum/1 -> x2/1
  x2/1 -> Out2/1, Mux/2, x1/1, Product/2  "x2"
  x1/1 -> Square/1, Sum/1, Out1/1, Mux/1  "x1"
  Mux/1 -> Scope/1
  Product/1 -> Mu/1
  Mu/1 -> Sum/2
  Square/1 -> Sum1/2
  Constant/1 -> Sum1/1
  Sum1/1 -> Product/1
  Constant1/1 -> Sum3/1
  Mux1/1 -> Scope1/1
  Product1/1 -> Mu1/1
  Mu1/1 -> Sum2/2
  Sum2/1 -> x4/1
  x3/1 -> Square1/1, Sum2/1, Out3/1, Mux1/1  "x1"
  Square1/1 -> Sum3/2
  Sum3/1 -> Product1/1
  x4/1 -> Out4/1, Mux1/2, x3/1, Product1/2  "x2"
  Constant2/1 -> Sum5/1
  Mux2/1 -> Scope2/1
  Product2/1 -> Mu2/1
  Sum4/1 -> x6/1
  x5/1 -> Square2/1, Sum4/1, Out5/1, Mux2/1  "x1"
  Square2/1 -> Sum5/2
  Sum5/1 -> Product2/1
  Sum7/1 -> Product3/1
  Mu2/1 -> Sum4/2
  x8/1 -> Out8/1, Mux3/2, x7/1, Product3/2  "x2"
  Square3/1 -> Sum7/2
  x6/1 -> Out6/1, Mux2/2, x5/1, Product2/2  "x2"
  x7/1 -> Square3/1, Sum6/1, Out7/1, Mux3/1  "x1"
  Mu3/1 -> Sum6/2
  Product3/1 -> Mu3/1
  Mux3/1 -> Scope3/1
  Sum6/1 -> x8/1
  Constant3/1 -> Sum7/1
  x10/1 -> Out10/1, Mux4/2, x9/1, Product4/2  "x2"
  Sum9/1 -> Product4/1
  Square4/1 -> Sum9/2
  Mu4/1 -> Sum8/2
  Sum8/1 -> x10/1
  x9/1 -> Square4/1, Sum8/1, Out9/1, Mux4/1  "x1"
  Product4/1 -> Mu4/1
  Constant4/1 -> Sum9/1
  Mux4/1 -> Scope4/1
  Sum18/1 -> x12/1
  x20/1 -> Square9/1, Sum18/1, Out19/1, Mux9/1  "x1"
  Constant9/1 -> Sum19/1
  Product9/1 -> Mu9/1
  Mu9/1 -> Sum18/2
  Square9/1 -> Sum19/2
  Sum19/1 -> Product9/1
  Mux9/1 -> Scope9/1
  x12/1 -> Out20/1, Mux9/2, x20/1, Product9/2  "x2"
  Constant8/1 -> Sum17/1
  x18/1 -> Square8/1, Sum16/1, Out17/1, Mux8/1  "x1"
  Sum16/1 -> x19/1
  Mux8/1 -> Scope8/1
  Mu8/1 -> Sum16/2
  Product8/1 -> Mu8/1
  Sum14/1 -> x17/1
  Mu7/1 -> Sum14/2
  Sum17/1 -> Product8/1
  x16/1 -> Square7/1, Sum14/1, Out15/1, Mux7/1  "x1"
  Mux7/1 -> Scope7/1
  Constant5/1 -> Sum11/1
  Mux5/1 -> Scope5/1
  Product5/1 -> Mu5/1
  Square7/1 -> Sum15/2
  Sum10/1 -> x13/1
  x11/1 -> Square5/1, Sum10/1, Out11/1, Mux5/1  "x1"
  Square5/1 -> Sum11/2
  Sum11/1 -> Product5/1
  Sum15/1 -> Product7/1
  Constant7/1 -> Sum15/1
  x19/1 -> Out18/1, Mux8/2, x18/1, Product8/2  "x2"
  Sum13/1 -> Product6/1
  Mu5/1 -> Sum10/2
  x15/1 -> Out14/1, Mux6/2, x14/1, Product6/2  "x2"
  Square6/1 -> Sum13/2
  x13/1 -> Out12/1, Mux5/2, x11/1, Product5/2  "x2"
  x14/1 -> Square6/1, Sum12/1, Out13/1, Mux6/1  "x1"
  Square8/1 -> Sum17/2
  Mu6/1 -> Sum12/2
  Product6/1 -> Mu6/1
  Mux6/1 -> Scope6/1
  x17/1 -> Out16/1, Mux7/2, x16/1, Product7/2  "x2"
  Sum12/1 -> x15/1
  Constant6/1 -> Sum13/1
  Product7/1 -> Mu7/1
  Sum38/1 -> x22/1
  Constant14/1 -> Sum39/1
  Product14/1 -> Mu14/1
  Mu14/1 -> Sum38/2
  Square14/1 -> Sum39/2
  Sum39/1 -> Product14/1
  x22/1 -> Out30/1, Mux14/2, x40/1, Product14/2  "x2"
  Product16/1 -> Mu16/1
  Mux16/1 -> Scope16/1
  Mu16/1 -> Sum24/2
  Square18/1 -> Sum29/2
  Product17/1 -> Mu17/1
  x26/1 -> Square16/1, Sum24/1, Out33/1, Mux16/1  "x1"
  x25/1 -> Out32/1, Mux15/2, x23/1, Product15/2  "x2"
  Mu15/1 -> Sum22/2
  Sum25/1 -> Product16/1
  x27/1 -> Out34/1, Mux16/2, x26/1, Product16/2  "x2"
  Square16/1 -> Sum25/2
  Constant17/1 -> Sum27/1
  Product15/1 -> Mu15/1
  Square15/1 -> Sum23/2
  Sum27/1 -> Product17/1
  x23/1 -> Square15/1, Sum22/1, Out31/1, Mux15/1  "x1"
  Mux15/1 -> Scope15/1
  Sum23/1 -> Product15/1
  Mux17/1 -> Scope17/1
  Mu17/1 -> Sum26/2
  Mux18/1 -> Scope18/1
  Mu18/1 -> Sum28/2
  x40/1 -> Square14/1, Sum38/1, Out29/1, Mux14/1  "x1"
  x28/1 -> Square17/1, Sum26/1, Out35/1, Mux17/1  "x1"
  Sum26/1 -> x29/1
  Sum29/1 -> Product18/1
  Product18/1 -> Mu18/1
  x24/1 -> Out40/1, Mux19/2, x33/1, Product19/2  "x2"
  Sum22/1 -> x25/1
  Sum28/1 -> x31/1
  x30/1 -> Square18/1, Sum28/1, Out37/1, Mux18/1  "x1"
  Sum24/1 -> x27/1
  Constant18/1 -> Sum29/1
  Sum31/1 -> Product19/1
  Mux14/1 -> Scope14/1
  Mu19/1 -> Sum30/2
  x33/1 -> Square19/1, Sum30/1, Out39/1, Mux19/1  "x1"
  x29/1 -> Out36/1, Mux17/2, x28/1, Product17/2  "x2"
  Sum30/1 -> x24/1
  Constant19/1 -> Sum31/1
  Product19/1 -> Mu19/1
  Mux19/1 -> Scope19/1
  Constant13/1 -> Sum37/1
  x38/1 -> Square13/1, Sum36/1, Out27/1, Mux13/1  "x1"
  Sum36/1 -> x39/1
  Mux13/1 -> Scope13/1
  Mu13/1 -> Sum36/2
  Product13/1 -> Mu13/1
  Square13/1 -> Sum37/2
  Square19/1 -> Sum31/2
  Sum34/1 -> x37/1
  Mu12/1 -> Sum34/2
  Sum37/1 -> Product13/1
  x36/1 -> Square12/1, Sum34/1, Out25/1, Mux12/1  "x1"
  Mux12/1 -> Scope12/1
  Constant10/1 -> Sum21/1
  x31/1 -> Out38/1, Mux18/2, x30/1, Product18/2  "x2"
  Mux10/1 -> Scope10/1
  Product10/1 -> Mu10/1
  Square12/1 -> Sum35/2
  Sum20/1 -> x32/1
  x21/1 -> Square10/1, Sum20/1, Out21/1, Mux10/1  "x1"
  Square10/1 -> Sum21/2
  Sum21/1 -> Product10/1
  Sum35/1 -> Product12/1
  Constant12/1 -> Sum35/1
  Constant15/1 -> Sum23/1
  x39/1 -> Out28/1, Mux13/2, x38/1, Product13/2  "x2"
  Sum33/1 -> Product11/1
  Mu10/1 -> Sum20/2
  x35/1 -> Out24/1, Mux11/2, x34/1, Product11/2  "x2"
  Square11/1 -> Sum33/2
  x32/1 -> Out22/1, Mux10/2, x21/1, Product10/2  "x2"
  x34/1 -> Square11/1, Sum32/1, Out23/1, Mux11/1  "x1"
  Mu11/1 -> Sum32/2
  Product11/1 -> Mu11/1
  Mux11/1 -> Scope11/1
  x37/1 -> Out26/1, Mux12/2, x36/1, Product12/2  "x2"
  Constant16/1 -> Sum25/1
  Sum32/1 -> x35/1
  Square17/1 -> Sum27/2
  Constant11/1 -> Sum33/1
  Product12/1 -> Mu12/1
  Square24/1 -> Sum69/2
  x65/1 -> Out78/1, Mux30/2, x64/1, Product30/2  "x2"
  Sum71/1 -> Product25/1
  Constant22/1 -> Sum54/1
  Mux24/1 -> Scope24/1
  Square31/1 -> Sum65/2
  Constant25/1 -> Sum71/1
  Mu25/1 -> Sum70/2
  Sum70/1 -> x73/1
  Mux31/1 -> Scope31/1
  x67/1 -> Square31/1, Sum64/1, Out79/1, Mux31/1  "x1"
  Constant31/1 -> Sum65/1
  Sum57/1 -> x60/1
  Square25/1 -> Sum71/2
  Sum65/1 -> Product31/1
  Mu31/1 -> Sum64/2
  Sum62/1 -> Product30/1
  x61/1 -> Square29/1, Sum59/1, Out75/1, Mux29/1  "x1"
  Sum59/1 -> x62/1
  x57/1 -> Out80/1, Mux31/2, x67/1, Product31/2  "x2"
  Mux29/1 -> Scope29/1
  Mu30/1 -> Sum61/2
  Mux30/1 -> Scope30/1
  Mu29/1 -> Sum59/2
  x75/1 -> Square26/1, Sum72/1, Out69/1, Mux26/1  "x1"
  Product27/1 -> Mu27/1
  Square28/1 -> Sum58/2
  Sum60/1 -> Product29/1
  x62/1 -> Out76/1, Mux29/2, x61/1, Product29/2  "x2"
  x60/1 -> Out74/1, Mux28/2, x59/1, Product28/2  "x2"
  Square27/1 -> Sum56/2
  Sum58/1 -> Product28/1
  Mu28/1 -> Sum57/2
  Sum64/1 -> x57/1
  Square26/1 -> Sum73/2
  Product29/1 -> Mu29/1
  Mux28/1 -> Scope28/1
  x55/1 -> Out70/1, Mux26/2, x75/1, Product26/2  "x2"
  Constant26/1 -> Sum73/1
  Product26/1 -> Mu26/1
  Sum53/1 -> x66/1
  Sum78/1 -> x42/1
  Constant34/1 -> Sum79/1
  Product34/1 -> Mu34/1
  Mu34/1 -> Sum78/2
  Square34/1 -> Sum79/2
  Sum79/1 -> Product34/1
  Product24/1 -> Mu24/1
  x71/1 -> Out66/1, Mux24/2, x70/1, Product24/2  "x2"
  Product31/1 -> Mu31/1
  Product23/1 -> Mu23/1
  Sum68/1 -> x71/1
  Mu23/1 -> Sum66/2
  Square29/1 -> Sum60/2
  Constant30/1 -> Sum62/1
  x66/1 -> Out62/1, Mux22/2, x54/1, Product22/2  "x2"
  Square23/1 -> Sum67/2
  x42/1 -> Out50/1, Mux34/2, x80/1, Product34/2  "x2"
  x68/1 -> Square23/1, Sum66/1, Out63/1, Mux23/1  "x1"
  Sum67/1 -> Product23/1
  Mu22/1 -> Sum53/2
  x73/1 -> Out68/1, Mux25/2, x72/1, Product25/2  "x2"
  x69/1 -> Out64/1, Mux23/2, x68/1, Product23/2  "x2"
  Mux27/1 -> Scope27/1
  Square22/1 -> Sum54/2
  Sum69/1 -> Product24/1
  x54/1 -> Square22/1, Sum53/1, Out61/1, Mux22/1  "x1"
  Constant24/1 -> Sum69/1
  Product36/1 -> Mu36/1
  Mux36/1 -> Scope36/1
  Product28/1 -> Mu28/1
  Constant28/1 -> Sum58/1
  Mu36/1 -> Sum44/2
  Square38/1 -> Sum49/2
  Product37/1 -> Mu37/1
  x70/1 -> Square24/1, Sum68/1, Out65/1, Mux24/1  "x1"
  x46/1 -> Square36/1, Sum44/1, Out53/1, Mux36/1  "x1"
  x45/1 -> Out52/1, Mux35/2, x43/1, Product35/2  "x2"
  Mu35/1 -> Sum42/2
  Product22/1 -> Mu22/1
  Constant29/1 -> Sum60/1
  Sum45/1 -> Product36/1
  x47/1 -> Out54/1, Mux36/2, x46/1, Product36/2  "x2"
  Square36/1 -> Sum45/2
  Constant37/1 -> Sum47/1
  Product35/1 -> Mu35/1
  Square35/1 -> Sum43/2
  Mux22/1 -> Scope22/1
  Sum47/1 -> Product37/1
  x43/1 -> Square35/1, Sum42/1, Out51/1, Mux35/1  "x1"
  Constant27/1 -> Sum56/1
  Mux35/1 -> Scope35/1
  Sum43/1 -> Product35/1
  Mux37/1 -> Scope37/1
  Mu37/1 -> Sum46/2
  Mux38/1 -> Scope38/1
  Mu38/1 -> Sum48/2
  x80/1 -> Square34/1, Sum78/1, Out49/1, Mux34/1  "x1"
  x48/1 -> Square37/1, Sum46/1, Out55/1, Mux37/1  "x1"
  Sum55/1 -> x58/1
  Sum46/1 -> x49/1
  Sum56/1 -> Product27/1
  Sum49/1 -> Product38/1
  Product38/1 -> Mu38/1
  x44/1 -> Out60/1, Mux39/2, x53/1, Product39/2  "x2"
  Sum42/1 -> x45/1
  Sum48/1 -> x51/1
  x50/1 -> Square38/1, Sum48/1, Out57/1, Mux38/1  "x1"
  Sum44/1 -> x47/1
  Constant38/1 -> Sum49/1
  Sum51/1 -> Product39/1
  Mux34/1 -> Scope34/1
  Sum61/1 -> x65/1
  Mu39/1 -> Sum50/2
  Mu26/1 -> Sum72/2
  x53/1 -> Square39/1, Sum50/1, Out59/1, Mux39/1  "x1"
  x49/1 -> Out56/1, Mux37/2, x48/1, Product37/2  "x2"
  Sum50/1 -> x44/1
  Constant39/1 -> Sum51/1
  Product39/1 -> Mu39/1
  Mux39/1 -> Scope39/1
  x59/1 -> Square28/1, Sum57/1, Out73/1, Mux28/1  "x1"
  Sum73/1 -> Product26/1
  Product30/1 -> Mu30/1
  x58/1 -> Out72/1, Mux27/2, x56/1, Product27/2  "x2"
  Constant33/1 -> Sum77/1
  x78/1 -> Square33/1, Sum76/1, Out47/1, Mux33/1  "x1"
  Sum76/1 -> x79/1
  Mux33/1 -> Scope33/1
  Mux25/1 -> Scope25/1
  Mu33/1 -> Sum76/2
  x64/1 -> Square30/1, Sum61/1, Out77/1, Mux30/1  "x1"
  Product33/1 -> Mu33/1
  Sum72/1 -> x55/1
  Mux26/1 -> Scope26/1
  Square33/1 -> Sum77/2
  x72/1 -> Square25/1, Sum70/1, Out67/1, Mux25/1  "x1"
  Square39/1 -> Sum51/2
  Sum74/1 -> x77/1
  Mu24/1 -> Sum68/2
  Constant23/1 -> Sum67/1
  Square30/1 -> Sum62/2
  Mu32/1 -> Sum74/2
  Sum77/1 -> Product33/1
  x76/1 -> Square32/1, Sum74/1, Out45/1, Mux32/1  "x1"
  Mux32/1 -> Scope32/1
  Constant20/1 -> Sum41/1
  x51/1 -> Out58/1, Mux38/2, x50/1, Product38/2  "x2"
  Sum54/1 -> Product22/1
  Mux23/1 -> Scope23/1
  Mux20/1 -> Scope20/1
  Product20/1 -> Mu20/1
  Square32/1 -> Sum75/2
  Sum40/1 -> x52/1
  x41/1 -> Square20/1, Sum40/1, Out41/1, Mux20/1  "x1"
  Square20/1 -> Sum41/2
  Sum41/1 -> Product20/1
  Sum75/1 -> Product32/1
  Sum66/1 -> x69/1
  Constant32/1 -> Sum75/1
  Constant35/1 -> Sum43/1
  x79/1 -> Out48/1, Mux33/2, x78/1, Product33/2  "x2"
  Sum63/1 -> Product21/1
  Mu20/1 -> Sum40/2
  x74/1 -> Out44/1, Mux21/2, x63/1, Product21/2  "x2"
  Mu27/1 -> Sum55/2
  Square21/1 -> Sum63/2
  Product25/1 -> Mu25/1
  x52/1 -> Out42/1, Mux20/2, x41/1, Product20/2  "x2"
  x56/1 -> Square27/1, Sum55/1, Out71/1, Mux27/1  "x1"
  x63/1 -> Square21/1, Sum52/1, Out43/1, Mux21/1  "x1"
  Mu21/1 -> Sum52/2
  Product21/1 -> Mu21/1
  Mux21/1 -> Scope21/1
  x77/1 -> Out46/1, Mux32/2, x76/1, Product32/2  "x2"
  Constant36/1 -> Sum45/1
  Sum52/1 -> x74/1
  Square37/1 -> Sum47/2
  Constant21/1 -> Sum63/1
  Product32/1 -> Mu32/1
  Sum92/1 -> x95/1
  Mux41/1 -> Scope41/1
  Sum81/1 -> Product40/1
  Square48/1 -> Sum89/2
  Constant41/1 -> Sum93/1
  Mu42/1 -> Sum94/2
  Mux44/1 -> Scope44/1
  Product43/1 -> Mu43/1
  Sum98/1 -> x82/1
  Mux43/1 -> Scope43/1
  x90/1 -> Square48/1, Sum88/1, Out97/1, Mux48/1  "x1"
  Sum99/1 -> Product44/1
  x86/1 -> Square46/1, Sum84/1, Out93/1, Mux46/1  "x1"
  x83/1 -> Square45/1, Sum82/1, Out91/1, Mux45/1  "x1"
  Constant45/1 -> Sum83/1
  Mux40/1 -> Scope40/1
  Product40/1 -> Mu40/1
  x96/1 -> Square42/1, Sum94/1, Out85/1, Mux42/1  "x1"
  x81/1 -> Square40/1, Sum80/1, Out81/1, Mux40/1  "x1"
  Product46/1 -> Mu46/1
  Constant46/1 -> Sum85/1
  Constant42/1 -> Sum95/1
  x99/1 -> Out88/1, Mux43/2, x98/1, Product43/2  "x2"
  Sum95/1 -> Product42/1
  Square40/1 -> Sum81/2
  Mu45/1 -> Sum82/2
  Mu40/1 -> Sum80/2
  Sum93/1 -> Product41/1
  x94/1 -> Square41/1, Sum92/1, Out83/1, Mux41/1  "x1"
  x92/1 -> Out82/1, Mux40/2, x81/1, Product40/2  "x2"
  Square41/1 -> Sum93/2
  Sum94/1 -> x97/1
  Mu41/1 -> Sum92/2
  Product41/1 -> Mu41/1
  Constant48/1 -> Sum89/1
  Square47/1 -> Sum87/2
  Mu44/1 -> Sum98/2
  Sum88/1 -> x91/1
  Sum83/1 -> Product45/1
  Mux49/1 -> Scope49/1
  Sum96/1 -> x99/1
  Mu43/1 -> Sum96/2
  Constant40/1 -> Sum81/1
  Product49/1 -> Mu49/1
  Product42/1 -> Mu42/1
  x97/1 -> Out86/1, Mux42/2, x96/1, Product42/2  "x2"
  Constant43/1 -> Sum97/1
  Square44/1 -> Sum99/2
  x98/1 -> Square43/1, Sum96/1, Out87/1, Mux43/1  "x1"
  Product44/1 -> Mu44/1
  Product47/1 -> Mu47/1
  x82/1 -> Out90/1, Mux44/2, x100/1, Product44/2  "x2"
  x91/1 -> Out98/1, Mux48/2, x90/1, Product48/2  "x2"
  Sum90/1 -> x84/1
  Sum85/1 -> Product46/1
  Mu46/1 -> Sum84/2
  Square45/1 -> Sum83/2
  x95/1 -> Out84/1, Mux41/2, x94/1, Product41/2  "x2"
  Mux42/1 -> Scope42/1
  Square46/1 -> Sum85/2
  Product45/1 -> Mu45/1
  Square49/1 -> Sum91/2
  x89/1 -> Out96/1, Mux47/2, x88/1, Product47/2  "x2"
  x87/1 -> Out94/1, Mux46/2, x86/1, Product46/2  "x2"
  Mux45/1 -> Scope45/1
  Sum87/1 -> Product47/1
  x100/1 -> Square44/1, Sum98/1, Out89/1, Mux44/1  "x1"
  Constant44/1 -> Sum99/1
  Sum80/1 -> x92/1
  Mu47/1 -> Sum86/2
  Product48/1 -> Mu48/1
  Mu48/1 -> Sum88/2
  Square42/1 -> Sum95/2
  Constant47/1 -> Sum87/1
  x88/1 -> Square47/1, Sum86/1, Out95/1, Mux47/1  "x1"
  x84/1 -> Out100/1, Mux49/2, x93/1, Product49/2  "x2"
  Mux47/1 -> Scope47/1
  Mux48/1 -> Scope48/1
  Sum84/1 -> x87/1
  Square43/1 -> Sum97/2
  Mux46/1 -> Scope46/1
  Sum89/1 -> Product48/1
  Sum82/1 -> x85/1
  x85/1 -> Out92/1, Mux45/2, x83/1, Product45/2  "x2"
  Mu49/1 -> Sum90/2
  Sum97/1 -> Product43/1
  Constant49/1 -> Sum91/1
  Sum86/1 -> x89/1
  x93/1 -> Square49/1, Sum90/1, Out99/1, Mux49/1  "x1"
  Sum91/1 -> Product49/1
  x194/1 -> Out199/1, Mux94/1, Square94/1, Sum190/1  "x1"
  Sum197/1 -> Product88/1
  Constant94/1 -> Sum191/1
  Mux93/1 -> Scope93/1
  Mux92/1 -> Scope92/1
  x184/1 -> Out200/1, Mux94/2, Product94/2, x194/1  "x2"
  Square87/1 -> Sum195/2
  Mu93/1 -> Sum187/2
  Constant89/1 -> Sum199/1
  x189/1 -> Out196/1, Mux92/2, Product92/2, x188/1  "x2"
  x187/1 -> Out194/1, Mux91/2, Product91/2, x186/1  "x2"
  Mux90/1 -> Scope90/1
  Mux87/1 -> Scope87/1
  x182/1 -> Out190/1, Mux89/2, Product89/2, x103/1  "x2"
  Sum190/1 -> x184/1
  Constant88/1 -> Sum197/1
  Square89/1 -> Sum199/2
  Product94/1 -> Mu94/1
  Mu88/1 -> Sum196/2
  Constant85/1 -> Sum180/1
  Sum196/1 -> x200/1
  Mux94/1 -> Scope94/1
  Mu86/1 -> Sum192/2
  Sum182/1 -> Product90/1
  x193/1 -> Out182/1, Mux85/2, Product85/2, x181/1  "x2"
  Sum187/1 -> x192/1
  Square85/1 -> Sum180/2
  Sum195/1 -> Product87/1
  x181/1 -> Out181/1, Mux85/1, Square85/1, Sum179/1  "x1"
  x200/1 -> Out188/1, Mux88/2, Product88/2, x199/1  "x2"
  Square94/1 -> Sum191/2
  Product85/1 -> Mu85/1
  x183/1 -> Out191/1, Mux90/1, Square90/1, Sum181/1  "x1"
  x191/1 -> Out197/1, Mux93/1, Square93/1, Sum187/1  "x1"
  Sum199/1 -> Product89/1
  Sum180/1 -> Product85/1
  Product88/1 -> Mu88/1
  Square93/1 -> Sum188/2
  Mux86/1 -> Scope86/1
  Product68/1 -> Mu68/1
  x149/1 -> Out142/1, Mux63/2, Product63/2, x137/1  "x2"
  Mu70/1 -> Sum151/2
  x173/1 -> Out144/1, Mux64/2, Product64/2, x161/1  "x2"
  Sum163/1 -> x167/1
  Constant79/1 -> Sum138/1
  Sum173/1 -> Product76/1
  Square76/1 -> Sum173/2
  Sum150/1 -> Product65/1
  Constant92/1 -> Sum186/1
  x175/1 -> Out145/1, Mux76/1, Square76/1, Sum172/1  "x1"
  Square74/1 -> Sum159/2
  Sum172/1 -> x176/1
  Square83/1 -> Sum147/2
  Constant66/1 -> Sum164/1
  Mu91/1 -> Sum183/2
  Mu67/1 -> Sum165/2
  Sum170/1 -> x152/1
  Mux68/1 -> Scope68/1
  x162/1 -> Out177/1, Mux74/1, Square74/1, Sum158/1  "x1"
  x153/1 -> Out171/1, Mux70/1, Square70/1, Sum151/1  "x1"
  Mu77/1 -> Sum174/2
  Sum171/1 -> Product69/1
  Product74/1 -> Mu74/1
  Constant80/1 -> Sum140/1
  Constant64/1 -> Sum160/1
  x197/1 -> Out185/1, Mux87/1, Square87/1, Sum194/1  "x1"
  Sum148/1 -> x173/1
  Product76/1 -> Mu76/1
  Square81/1 -> Sum142/2
  Mu87/1 -> Sum194/2
  Product64/1 -> Mu64/1
  x161/1 -> Out143/1, Mux64/1, Square64/1, Sum148/1  "x1"
  Mu76/1 -> Sum172/2
  Square88/1 -> Sum197/2
  Mux81/1 -> Scope81/1
  Constant70/1 -> Sum152/1
  x139/1 -> Out151/1, Mux79/1, Square79/1, Sum137/1  "x1"
  Square80/1 -> Sum140/2
  x143/1 -> Out154/1, Mux80/2, Product80/2, x142/1  "x2"
  Sum142/1 -> Product81/1
  Square79/1 -> Sum138/2
  x141/1 -> Out152/1, Mux79/2, Product79/2, x139/1  "x2"
  Sum140/1 -> Product80/1
  Constant72/1 -> Sum157/1
  Mu79/1 -> Sum137/2
  x196/1 -> Out184/1, Mux86/2, Product86/2, x195/1  "x2"
  Mux77/1 -> Scope77/1
  x169/1 -> Out165/1, Mux67/1, Square67/1, Sum165/1  "x1"
  x142/1 -> Out153/1, Mux80/1, Square80/1, Sum139/1  "x1"
  Product81/1 -> Mu81/1
  x151/1 -> Out161/1, Mux65/1, Square65/1, Sum149/1  "x1"
  Product71/1 -> Mu71/1
  Product80/1 -> Mu80/1
  Mu80/1 -> Sum139/2
  Square82/1 -> Sum144/2
  Constant71/1 -> Sum154/1
  Mux80/1 -> Scope80/1
  Sum138/1 -> Product79/1
  Constant67/1 -> Sum166/1
  Mux70/1 -> Scope70/1
  x172/1 -> Out168/1, Mux68/2, Product68/2, x171/1  "x2"
  Mux64/1 -> Scope64/1
  Sum166/1 -> Product67/1
  Square65/1 -> Sum150/2
  Mu65/1 -> Sum149/2
  Sum191/1 -> Product94/1
  Mux82/1 -> Scope82/1
  Sum164/1 -> Product66/1
  Constant87/1 -> Sum195/1
  x166/1 -> Out163/1, Mux66/1, Square66/1, Sum163/1  "x1"
  x164/1 -> Out162/1, Mux65/2, Product65/2, x151/1  "x2"
  Sum165/1 -> x170/1
  Mu94/1 -> Sum190/2
  Mu66/1 -> Sum163/2
  Square72/1 -> Sum157/2
  Square64/1 -> Sum160/2
  Sum179/1 -> x193/1
  Product93/1 -> Mu93/1
  Sum146/1 -> x140/1
  Product83/1 -> Mu83/1
  Sum139/1 -> x143/1
  Mu69/1 -> Sum170/2
  Sum158/1 -> x163/1
  Constant82/1 -> Sum144/1
  Mux78/1 -> Scope78/1
  Square92/1 -> Sum186/2
  x140/1 -> Out160/1, Mux83/2, Product83/2, x150/1  "x2"
  Product82/1 -> Mu82/1
  Sum143/1 -> x148/1
  Sum144/1 -> Product82/1
  Sum152/1 -> Product70/1
  Sum141/1 -> x145/1
  Mux69/1 -> Scope69/1
  Square54/1 -> Sum129/2
  x126/1 -> Out138/1, Mux60/2, x125/1, Product60/2  "x2"
  Sum131/1 -> Product55/1
  Constant52/1 -> Sum114/1
  Mux54/1 -> Scope54/1
  Square55/1 -> Sum131/2
  Product55/1 -> Mu55/1
  Sum130/1 -> x134/1
  Mux61/1 -> Scope61/1
  Sum181/1 -> x185/1
  Sum188/1 -> Product93/1
  Product61/1 -> Mu61/1
  x147/1 -> Out157/1, Mux82/1, Square82/1, Sum143/1  "x1"
  Sum125/1 -> Product61/1
  Mu61/1 -> Sum124/2
  Sum122/1 -> Product60/1
  x122/1 -> Square59/1, Sum119/1, Out135/1, Mux59/1  "x1"
  Sum119/1 -> x123/1
  Mux89/1 -> Scope89/1
  Mux59/1 -> Scope59/1
  Mu60/1 -> Sum121/2
  x150/1 -> Out159/1, Mux83/1, Square83/1, Sum146/1  "x1"
  Mu59/1 -> Sum119/2
  x136/1 -> Square56/1, Sum132/1, Out129/1, Mux56/1  "x1"
  Product57/1 -> Mu57/1
  Square58/1 -> Sum118/2
  Mux63/1 -> Scope63/1
  Sum120/1 -> Product59/1
  Mux65/1 -> Scope65/1
  Mux83/1 -> Scope83/1
  x123/1 -> Out136/1, Mux59/2, x122/1, Product59/2  "x2"
  x121/1 -> Out134/1, Mux58/2, x120/1, Product58/2  "x2"
  Square57/1 -> Sum116/2
  Constant83/1 -> Sum147/1
  Sum118/1 -> Product58/1
  Mu58/1 -> Sum117/2
  Sum124/1 -> x118/1
  Product59/1 -> Mu59/1
  Mux58/1 -> Scope58/1
  Sum133/1 -> Product56/1
  Sum194/1 -> x198/1
  Constant56/1 -> Sum133/1
  Product56/1 -> Mu56/1
  Sum113/1 -> x127/1
  Sum178/1 -> x102/1
  Product84/1 -> Mu84/1
  Mu84/1 -> Sum178/2
  Square84/1 -> Sum189/2
  Mux76/1 -> Scope76/1
  Sum189/1 -> Product84/1
  x199/1 -> Out187/1, Mux88/1, Square88/1, Sum196/1  "x1"
  x102/1 -> Out110/1, Mux84/2, x190/1, Product84/2  "x2"
  Mux75/1 -> Scope75/1
  Mu68/1 -> Sum168/2
  Square56/1 -> Sum133/2
  Mu83/1 -> Sum146/2
  Constant65/1 -> Sum150/1
  x116/1 -> Out130/1, Mux56/2, x136/1, Product56/2  "x2"
  Sum177/1 -> Product78/1
  Product67/1 -> Mu67/1
  x170/1 -> Out166/1, Mux67/2, Product67/2, x169/1  "x2"
  x137/1 -> Out141/1, Mux63/1, Square63/1, Sum135/1  "x1"
  Mux60/1 -> Scope60/1
  Sum136/1 -> Product63/1
  Square78/1 -> Sum177/2
  Constant76/1 -> Sum173/1
  Constant68/1 -> Sum169/1
  Square69/1 -> Sum171/2
  Sum147/1 -> Product83/1
  x171/1 -> Out167/1, Mux68/1, Square68/1, Sum168/1  "x1"
  Sum176/1 -> x138/1
  Product69/1 -> Mu69/1
  Product72/1 -> Mu72/1
  Mu55/1 -> Sum130/2
  Sum154/1 -> Product71/1
  Mu71/1 -> Sum153/2
  Square70/1 -> Sum152/2
  Constant61/1 -> Sum125/1
  Square86/1 -> Sum193/2
  Product70/1 -> Mu70/1
  Square75/1 -> Sum162/2
  x160/1 -> Out176/1, Mux72/2, Product72/2, x159/1  "x2"
  Sum157/1 -> Product72/1
  Constant69/1 -> Sum171/1
  x103/1 -> Out189/1, Mux89/1, Square89/1, Sum198/1  "x1"
  Sum117/1 -> x121/1
  x198/1 -> Out186/1, Mux87/2, Product87/2, x197/1  "x2"
  Mu72/1 -> Sum155/2
  x145/1 -> Out156/1, Mux81/2, Product81/2, x144/1  "x2"
  Product92/1 -> Mu92/1
  Mux79/1 -> Scope79/1
  Mu74/1 -> Sum158/2
  Square67/1 -> Sum166/2
  x159/1 -> Out175/1, Mux72/1, Square72/1, Sum155/1  "x1"
  Square61/1 -> Sum125/2
  x154/1 -> Out180/1, Mux75/2, Product75/2, x165/1  "x2"
  x138/1 -> Out150/1, Mux78/2, Product78/2, x180/1  "x2"
  Mux72/1 -> Scope72/1
  Mux74/1 -> Scope74/1
  Sum153/1 -> x158/1
  Sum137/1 -> x141/1
  Square68/1 -> Sum169/2
  Mux71/1 -> Scope71/1
  Sum159/1 -> Product74/1
  Constant75/1 -> Sum162/1
  x128/1 -> Square61/1, Sum124/1, Out139/1, Mux61/1  "x1"
  Sum162/1 -> Product75/1
  x174/1 -> Out169/1, Mux69/1, Square69/1, Sum170/1  "x1"
  Product54/1 -> Mu54/1
  x132/1 -> Out126/1, Mux54/2, x131/1, Product54/2  "x2"
  Product53/1 -> Mu53/1
  Sum128/1 -> x132/1
  Product79/1 -> Mu79/1
  Mu53/1 -> Sum126/2
  Square59/1 -> Sum120/2
  Constant60/1 -> Sum122/1
  x127/1 -> Out122/1, Mux52/2, x115/1, Product52/2  "x2"
  Constant91/1 -> Sum184/1
  Square53/1 -> Sum127/2
  x129/1 -> Square53/1, Sum126/1, Out123/1, Mux53/1  "x1"
  Sum127/1 -> Product53/1
  x176/1 -> Out146/1, Mux76/2, Product76/2, x175/1  "x2"
  Mu52/1 -> Sum113/2
  Sum168/1 -> x172/1
  x134/1 -> Out128/1, Mux55/2, x133/1, Product55/2  "x2"
  x130/1 -> Out124/1, Mux53/2, x129/1, Product53/2  "x2"
  Mux57/1 -> Scope57/1
  Sum129/1 -> Product54/1
  Square77/1 -> Sum175/2
  Square63/1 -> Sum136/2
  x115/1 -> Square52/1, Sum113/1, Out121/1, Mux52/1  "x1"
  Mux66/1 -> Scope66/1
  Constant54/1 -> Sum129/1
  Sum135/1 -> x149/1
  Product90/1 -> Mu90/1
  Constant90/1 -> Sum182/1
  Product96/1 -> Mu96/1
  x188/1 -> Out195/1, Mux92/1, Square92/1, Sum185/1  "x1"
  Product58/1 -> Mu58/1
  Mux96/1 -> Scope96/1
  Constant58/1 -> Sum118/1
  Mu64/1 -> Sum148/2
  Mu96/1 -> Sum104/2
  Square98/1 -> Sum109/2
  Product97/1 -> Mu97/1
  x131/1 -> Square54/1, Sum128/1, Out125/1, Mux54/1  "x1"
  x107/1 -> Square96/1, Sum104/1, Out113/1, Mux96/1  "x1"
  Mu81/1 -> Sum141/2
  Square90/1 -> Sum182/2
  Sum160/1 -> Product64/1
  x106/1 -> Out112/1, Mux95/2, x104/1, Product95/2  "x2"
  Mu95/1 -> Sum102/2
  Product52/1 -> Mu52/1
  x178/1 -> Out148/1, Mux77/2, Product77/2, x177/1  "x2"
  Mu75/1 -> Sum161/2
  Sum169/1 -> Product68/1
  Constant59/1 -> Sum120/1
  Square71/1 -> Sum154/2
  Sum105/1 -> Product96/1
  Mu63/1 -> Sum135/2
  x167/1 -> Out164/1, Mux66/2, Product66/2, x166/1  "x2"
  Product75/1 -> Mu75/1
  x108/1 -> Out114/1, Mux96/2, x107/1, Product96/2  "x2"
  Constant97/1 -> Sum107/1
  Sum161/1 -> x154/1
  Product95/1 -> Mu95/1
  Sum107/1 -> Product97/1
  x104/1 -> Square95/1, Sum102/1, Out111/1, Mux95/1  "x1"
  x148/1 -> Out158/1, Mux82/2, Product82/2, x147/1  "x2"
  Constant57/1 -> Sum116/1
  Mux95/1 -> Scope95/1
  Sum103/1 -> Product95/1
  Constant78/1 -> Sum177/1
  Mux91/1 -> Scope91/1
  Mux97/1 -> Scope97/1
  Mu97/1 -> Sum106/2
  Constant63/1 -> Sum136/1
  Mux98/1 -> Scope98/1
  Mu98/1 -> Sum108/2
  x190/1 -> Square84/1, Sum178/1, Out109/1, Mux84/1  "x1"
  x109/1 -> Square97/1, Sum106/1, Out115/1, Mux97/1  "x1"
  Sum115/1 -> x119/1
  Sum183/1 -> x187/1
  Sum106/1 -> x110/1
  Sum116/1 -> Product57/1
  Sum109/1 -> Product98/1
  Product98/1 -> Mu98/1
  x105/1 -> Out120/1, Mux99/2, x114/1, Product99/2  "x2"
  Sum175/1 -> Product77/1
  Sum102/1 -> x106/1
  Sum108/1 -> x112/1
  Square66/1 -> Sum164/2
  x111/1 -> Square98/1, Sum108/1, Out117/1, Mux98/1  "x1"
  Sum104/1 -> x108/1
  Sum149/1 -> x164/1
  Constant98/1 -> Sum109/1
  x155/1 -> Out172/1, Mux70/2, Product70/2, x153/1  "x2"
  Sum151/1 -> x155/1
  Mux84/1 -> Scope84/1
  Sum111/1 -> Product99/1
  Sum121/1 -> x126/1
  Mu99/1 -> Sum110/2
  Sum192/1 -> x196/1
  Mu56/1 -> Sum132/2
  x114/1 -> Square99/1, Sum110/1, Out119/1, Mux99/1  "x1"
  x110/1 -> Out116/1, Mux97/2, x109/1, Product97/2  "x2"
  Constant86/1 -> Sum193/1
  Product66/1 -> Mu66/1
  Sum110/1 -> x105/1
  Constant99/1 -> Sum111/1
  Product99/1 -> Mu99/1
  x120/1 -> Square58/1, Sum117/1, Out133/1, Mux58/1  "x1"
  Product60/1 -> Mu60/1
  Constant73/1 -> Sum167/1
  x168/1 -> Square73/1, Sum156/1, Out107/1, Mux73/1  "x1"
  Sum156/1 -> x179/1
  Mux73/1 -> Scope73/1
  Mux55/1 -> Scope55/1
  Product63/1 -> Mu63/1
  Mu73/1 -> Sum156/2
  x125/1 -> Square60/1, Sum121/1, Out137/1, Mux60/1  "x1"
  Sum132/1 -> x116/1
  x157/1 -> Out106/1, Mux62/2, x146/1, Product62/2  "x2"
  Mux56/1 -> Scope56/1
  Sum193/1 -> Product86/1
  Product78/1 -> Mu78/1
  Square99/1 -> Sum111/2
  Sum155/1 -> x160/1
  x186/1 -> Out193/1, Mux91/1, Square91/1, Sum183/1  "x1"
  Square73/1 -> Sum167/2
  x133/1 -> Square55/1, Sum130/1, Out127/1, Mux55/1  "x1"
  Mux85/1 -> Scope85/1
  x152/1 -> Out170/1, Mux69/2, Product69/2, x174/1  "x2"
  Product62/1 -> Mu62/1
  x163/1 -> Out178/1, Mux74/2, Product74/2, x162/1  "x2"
  Sum134/1 -> x157/1
  Square62/1 -> Sum145/2
  Mu54/1 -> Sum128/2
  Constant53/1 -> Sum127/1
  Square60/1 -> Sum122/2
  Mu62/1 -> Sum134/2
  Mux67/1 -> Scope67/1
  Sum126/1 -> x130/1
  Product87/1 -> Mu87/1
  Sum145/1 -> Product62/1
  x185/1 -> Out192/1, Mux90/2, Product90/2, x183/1  "x2"
  Sum167/1 -> Product73/1
  x146/1 -> Square62/1, Sum134/1, Out105/1, Mux62/1  "x1"
  Constant62/1 -> Sum145/1
  Square91/1 -> Sum184/2
  Sum101/1 -> Product50/1
  Sum114/1 -> Product52/1
  Constant50/1 -> Sum101/1
  x112/1 -> Out118/1, Mux98/2, x111/1, Product98/2  "x2"
  Mux53/1 -> Scope53/1
  Mux50/1 -> Scope50/1
  Product50/1 -> Mu50/1
  Mu50/1 -> Sum100/2
  Sum186/1 -> Product92/1
  Sum100/1 -> x113/1
  x101/1 -> Square50/1, Sum100/1, Out101/1, Mux50/1  "x1"
  Sum185/1 -> x189/1
  Constant77/1 -> Sum175/1
  Product86/1 -> Mu86/1
  Constant55/1 -> Sum131/1
  Sum184/1 -> Product91/1
  Sum198/1 -> x182/1
  x195/1 -> Out183/1, Mux86/1, Square86/1, Sum192/1  "x1"
  x180/1 -> Out149/1, Mux78/1, Square78/1, Sum176/1  "x1"
  Constant81/1 -> Sum142/1
  Square50/1 -> Sum101/2
  Mu78/1 -> Sum176/2
  x144/1 -> Out155/1, Mux81/1, Square81/1, Sum141/1  "x1"
  Sum123/1 -> Product51/1
  Mu92/1 -> Sum185/2
  Mu82/1 -> Sum143/2
  x135/1 -> Out104/1, Mux51/2, x124/1, Product51/2  "x2"
  Mu57/1 -> Sum115/2
  Square51/1 -> Sum123/2
  x192/1 -> Out198/1, Mux93/2, Product93/2, x191/1  "x2"
  Mux88/1 -> Scope88/1
  x113/1 -> Out102/1, Mux50/2, x101/1, Product50/2  "x2"
  x117/1 -> Square57/1, Sum115/1, Out131/1, Mux57/1  "x1"
  x156/1 -> Out173/1, Mux71/1, Square71/1, Sum153/1  "x1"
  x124/1 -> Square51/1, Sum112/1, Out103/1, Mux51/1  "x1"
  x158/1 -> Out174/1, Mux71/2, Product71/2, x156/1  "x2"
  Mu51/1 -> Sum112/2
  Square95/1 -> Sum103/2
  Mux52/1 -> Scope52/1
  Product91/1 -> Mu91/1
  Mux51/1 -> Scope51/1
  Product77/1 -> Mu77/1
  Constant96/1 -> Sum105/1
  Mux99/1 -> Scope99/1
  Product73/1 -> Mu73/1
  Sum112/1 -> x135/1
  Square97/1 -> Sum107/2
  Mu85/1 -> Sum179/2
  x179/1 -> Out108/1, Mux73/2, x168/1, Product73/2  "x2"
  x165/1 -> Out179/1, Mux75/1, Square75/1, Sum161/1  "x1"
  x177/1 -> Out147/1, Mux77/1, Square77/1, Sum174/1  "x1"
  Constant95/1 -> Sum103/1
  Square52/1 -> Sum114/2
  Constant74/1 -> Sum159/1
  Product51/1 -> Mu51/1
  x118/1 -> Out140/1, Mux61/2, x128/1, Product61/2  "x2"
  x119/1 -> Out132/1, Mux57/2, x117/1, Product57/2  "x2"
  Mu90/1 -> Sum181/2
  Constant51/1 -> Sum123/1
  Constant84/1 -> Sum189/1
  Sum174/1 -> x178/1
  Constant93/1 -> Sum188/1
  Mu89/1 -> Sum198/2
  Product65/1 -> Mu65/1
  Mux62/1 -> Scope62/1
  Product89/1 -> Mu89/1
  Square96/1 -> Sum105/2
